simulink model "P1Q5"  (R2017a)
settings: Solver=VariableStepAuto  StartTime=0.0  StopTime=0.3  RelTol=1e-3
settings Model: Creator=ifaruk  LastModifiedBy=ifaruk

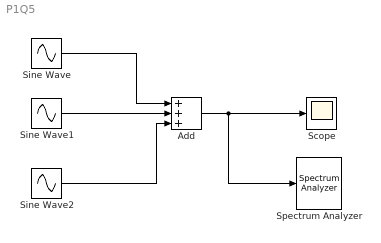
== system P1Q5 ==
  Add : Sum  Inputs=+++
  Scope : Scope
  Sine Wave : Sin  SineType=Sample based  Amplitude=0.5  Samples=1000  SampleTime=0.0001
  Sine Wave1 : Sin  SineType=Sample based  Amplitude=2  Frequency=5000  Samples=500  SampleTime=0.0001
  Sine Wave2 : Sin  SineType=Sample based  Amplitude=1.5  Samples=100  SampleTime=0.0001
  Spectrum Analyzer : SpectrumAnalyzer
  wires:
  Sine Wave/1 -> Add/1
  Sine Wave1/1 -> Add/2
  Sine Wave2/1 -> Add/3
  Add/1 -> Spectrum Analyzer/1, Scope/1
